simulink model "ext_steer_all"  (Simulink 7.6)
settings: Solver=ode45  SolverMode=SingleTasking  StartTime=0  StopTime=110  FixedStep=0.002  RelTol=1e-3  AbsTol=1e-6
libraries: Solver_SF x1
settings Model: Creator=ywata  LastModifiedBy=hkawanishi  ExtModeTrigMode=oneshot  ExtModeArmWhenConnect=off
settings DataIOCC: LimitDataPoints=off  SignalLoggingName=sigsOut
settings OptimizationCC: BlockReduction=off  BooleanDataType=off  ExpressionDepthLimit=128
settings DebuggingCC: SaveWithParameterizedLinksMsg=none  SignalResolutionControl=TryResolveAllWithWarning  SolverPrmCheckMsg=none  MultiTaskDSMMsg=warning  MultiTaskCondExecSysMsg=none
settings HardwareCC: TargetUnknown=on
settings RTWCC: TemplateMakefile=grt_vc.tmf  IncludeERTFirstTime=on
settings CodeAppCC: CustomSymbolStrType=$N$R$M_T
settings GRTTargetCC: TargetFcnLib=ansi_tfl_tmw.mat

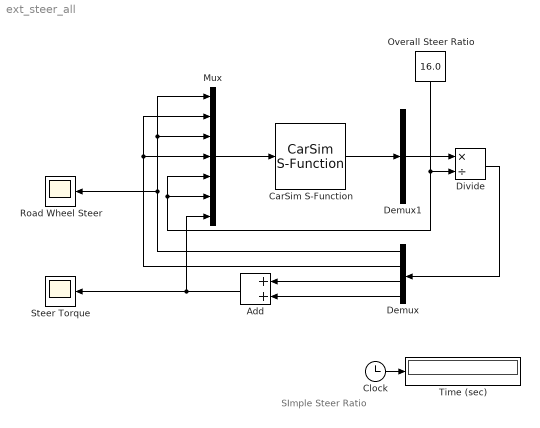
== system ext_steer_all ==
  note: SImple Steer Ratio
  Add : Sum
  CarSim S-Function : Solver_SF/CarSim S-Function  Priority=1  SIMFILE=simfile.sim
  Clock : Clock
      settings: Decimation=10
  Demux : Demux
  Demux1 : Demux  Outputs=[4]
  Divide : Product  Inputs=*/
  Mux : Mux  Inputs=7
  Overall Steer Ratio : Constant  Value=16.0
  Road Wheel Steer : Scope
      settings: TickLabels=on  TimeRange=7  YMin=-2  YMax=1  DataFormat=Array  SampleTime=100
  Steer Torque : Scope
      settings: TickLabels=on  TimeRange=7  DataFormat=Array  SampleTime=100
  Time (sec) : Display
      settings: Format=bank  Decimation=100
  wires:
  Clock/1 -> Time (sec)/1
  Demux1/1 -> Divide/1
  Divide/1 -> Demux/1
  Demux/1 -> Mux/3, Mux/1, Road Wheel Steer/1
  Demux/2 -> Mux/4, Mux/2
  Overall Steer Ratio/1 -> Divide/2, Mux/6, Mux/5
  Demux/3 -> Add/1
  Demux/4 -> Add/2
  Add/1 -> Steer Torque/1, Mux/7
  CarSim S-Function/1 -> Demux1/1
  Mux/1 -> CarSim S-Function/1
